simulink model "simulation"  (R2018b)
settings: Solver=ode4  StartTime=0.0  StopTime=200  FixedStep=0.001  RelTol=1e-3
model workspace: external: MAT-File Y:\Aerospace\AeroSpace 4\Term 2\AutoPilot (Dr. Osama Saaid)\Tasks\Task 7\code\Non-Linear Simulation\AC_data.mat (data not in the file)
values from neighbouring files (symbols this model uses):
  stability_matrix = [-0.0415 0 -0.162 0 -0.00076 0 0 -0.338 0 0 0 0 ... (72 elements, 6x12)]    [AC_data.mat]
undefined symbols (not defined in the file or in its folder): plane, rotationVectorToMatrix, servo
libraries: simulink_extras x12, cstblocks x3, shared6dof x1, dspsigops x1
settings Model: Creator=OWNER  LastModifiedBy=OWNER

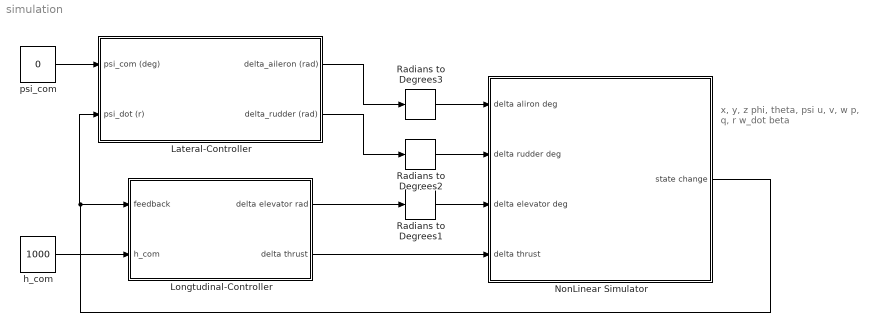
== system simulation ==
  note: x, y, z
      |
      | phi, theta, psi
      |
      | u, v, w
      |
      | p, q, r
      |
      | w_dot
      |
      | beta
  Lateral-Controller : Subsystem
  Longtudinal-Controller : Subsystem
  NonLinear Simulator : Subsystem
  Radians to Degrees1 : simulink_extras/Transformations/Radians to Degrees
  Radians to Degrees2 : simulink_extras/Transformations/Radians to Degrees
  Radians to Degrees3 : simulink_extras/Transformations/Radians to Degrees
  h_com : Constant  Value=1000
  psi_com : Constant  Value=0
  wires:
  Radians to Degrees3/1 -> NonLinear Simulator/1(delta aliron deg)
  Radians to Degrees2/1 -> NonLinear Simulator/2(delta rudder deg)
  Radians to Degrees1/1 -> NonLinear Simulator/3(delta elevator deg)
  h_com/1 -> Longtudinal-Controller/2(h_com)
  Longtudinal-Controller/1(delta elevator rad) -> Radians to Degrees1/1
  Longtudinal-Controller/2(delta thrust) -> NonLinear Simulator/4(delta thrust)
  psi_com/1 -> Lateral-Controller/1(psi_com (deg))
  Lateral-Controller/1(delta_aileron (rad)) -> Radians to Degrees3/1
  Lateral-Controller/2(delta_rudder (rad)) -> Radians to Degrees2/1
  NonLinear Simulator/1(state change) -> Lateral-Controller/2(psi_dot (r)), Longtudinal-Controller/1(feedback)

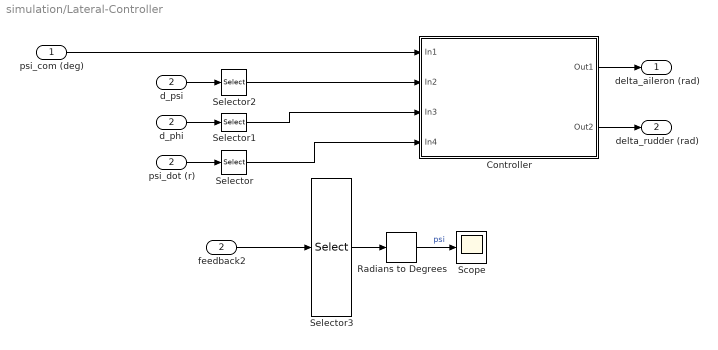
== system simulation/Lateral-Controller ==
  psi_com (deg) : Inport
  psi_dot (r) : Inport  Port=2
  Controller : Subsystem
  Radians to Degrees : simulink_extras/Transformations/Radians to Degrees
  Scope : Scope
  Selector : Selector  InputPortWidth=14  IndexOptions=Index vector (dialog)  Indices=[12]  OutputSizes=1
  Selector1 : Selector  InputPortWidth=14  IndexOptions=Index vector (dialog)  Indices=[4]  OutputSizes=1
  Selector2 : Selector  InputPortWidth=14  IndexOptions=Index vector (dialog)  Indices=[6]  OutputSizes=1
  Selector3 : Selector  InputPortWidth=14  IndexOptions=Index vector (dialog)  Indices=[6]  OutputSizes=1
  d_phi : InportShadow  Port=2
  d_psi : InportShadow  Port=2
  feedback2 : InportShadow  Port=2
  delta_aileron (rad) : Outport  VectorParamsAs1DForOutWhenUnconnected=on
  delta_rudder (rad) : Outport  Port=2  VectorParamsAs1DForOutWhenUnconnected=on
  wires:
  psi_com (deg)/1 -> Controller/1(In1)
  d_psi/1 -> Selector2/1
  d_phi/1 -> Selector1/1
  psi_dot (r)/1 -> Selector/1
  Controller/1(Out1) -> delta_aileron (rad)/1
  Controller/2(Out2) -> delta_rudder (rad)/1
  Selector3/1 -> Radians to Degrees/1
  feedback2/1 -> Selector3/1
  Radians to Degrees/1 -> Scope/1  "psi"
  Selector2/1 -> Controller/2(In2)
  Selector1/1 -> Controller/3(In3)
  Selector/1 -> Controller/4(In4)

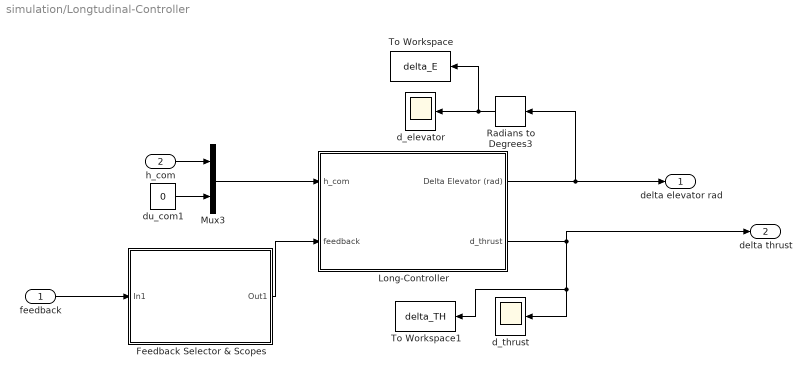
== system simulation/Longtudinal-Controller ==
  feedback : Inport
  h_com : Inport  Port=2
  Feedback Selector & Scopes : Subsystem
  "Long-Controller " : Subsystem
  Mux3 : Mux  Inputs=2
  Radians to Degrees3 : simulink_extras/Transformations/Radians to Degrees
  To Workspace : ToWorkspace  VariableName=delta_E  SaveFormat=Timeseries  SampleTime=-1
  To Workspace1 : ToWorkspace  VariableName=delta_TH  SaveFormat=Timeseries  SampleTime=-1
  d_elevator : Scope
  d_thrust : Scope
  du_com1 : Constant  Value=0
  delta elevator rad : Outport
  delta thrust : Outport  Port=2
  wires:
  Feedback Selector & Scopes/1(Out1) -> "Long-Controller "/2(feedback)
  Mux3/1 -> "Long-Controller "/1(h_com)
  h_com/1 -> Mux3/1
  du_com1/1 -> Mux3/2
  "Long-Controller "/1(Delta Elevator (rad)) -> delta elevator rad/1, Radians to Degrees3/1
  feedback/1 -> Feedback Selector & Scopes/1(In1)
  Radians to Degrees3/1 -> To Workspace/1, d_elevator/1
  "Long-Controller "/2(d_thrust) -> delta thrust/1, To Workspace1/1, d_thrust/1

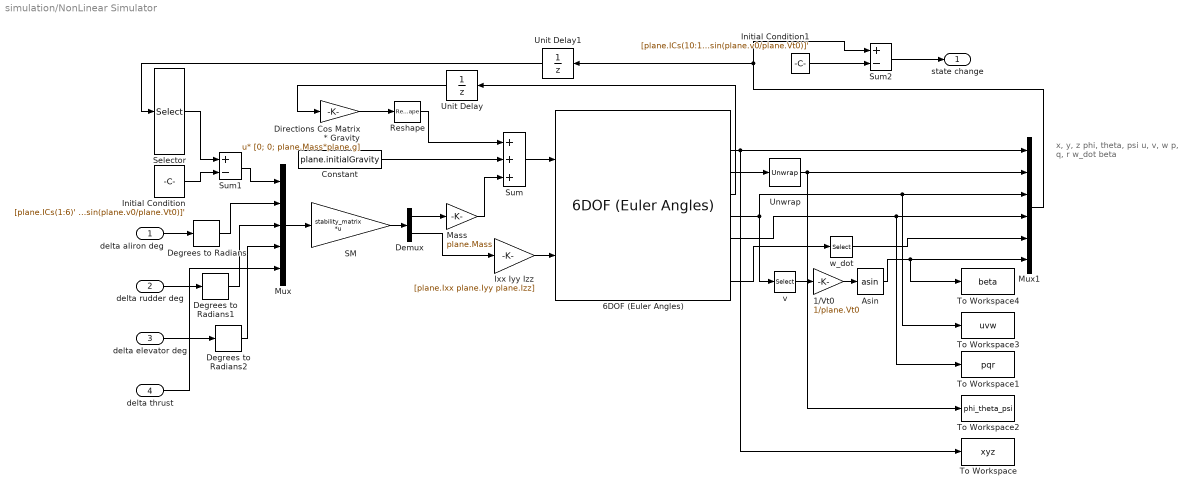
== system simulation/NonLinear Simulator ==
  note: x, y, z
      |
      | phi, theta, psi
      |
      | u, v, w
      |
      | p, q, r
      |
      | w_dot
      |
      | beta
  delta aliron deg : Inport
  delta rudder deg : Inport  Port=2
  delta elevator deg : Inport  Port=3
  delta thrust : Inport  Port=4
  1/Vt0 : Gain  Gain=1/plane.Vt0
  6DOF (Euler Angles) : shared6dof/6DOF (Euler Angles)  units=English (Velocity in ft/s)  mtype=Fixed  rep=Euler Angles  xme_0=[plane.ICs(10:12) ]'  Vm_0=[plane.ICs(1:3)]'  eul_0=[plane.ICs(7:9)]'  pm_0=[plane.ICs(4:6)]'  mass_0=plane.Mass  mass_e=0.5  mass_f=2.0  inertia=plane.I  inertia_e=eye(3)  inertia_f=2*eye(3)  k_quat=1.0  vre_flag=on  abi_flag=off  aMode=0  xme_statename=''  Vm_statename=''  eul_statename=''  quat_statename=''  pm_statename=''  mass_statename=''
      settings: SourceProductBaseCode=AE
  Asin : Trigonometry  Operator=asin
  Constant : Constant  Value=plane.initialGravity
  Degrees to Radians : simulink_extras/Transformations/Degrees to Radians
  Degrees to Radians1 : simulink_extras/Transformations/Degrees to Radians
  Degrees to Radians2 : simulink_extras/Transformations/Degrees to Radians
  Demux : Demux  Outputs=2
  Directions Cos Matrix * Gravity : Gain  Gain=[0; 0; plane.Mass*plane.g]  Multiplication=Matrix(u*K)
  Initial Condition : Constant  Value=[plane.ICs(1:6)' plane.ICs_dot0(3)' asin(plane.v0/plane.Vt0)]'
  Initial Condition1 : Constant  Value="[plane.ICs(10:12)' plane.ICs(7:9)' plane.ICs(1:6)'  plane.ICs_dot0(3)' asin(plane.v0/plane.Vt0)]'"
  Ixx Iyy Izz : Gain  Gain=[plane.Ixx plane.Iyy plane.Izz]
  "Mass " : Gain  Gain=plane.Mass
  Mux : Mux  Inputs=5
  Mux1 : Mux  Inputs=6
  Reshape : Reshape
  SM : Gain  Gain=stability_matrix  Multiplication=Matrix(K*u) (u vector)
  Selector : Selector  InputPortWidth=14  IndexOptions=Index vector (dialog)  Indices=[7:14]  OutputSizes=1
  Sum : Sum  Inputs=+++
  Sum1 : Sum  Inputs=+-
  Sum2 : Sum  Inputs=+-
  To Workspace : ToWorkspace  VariableName=xyz  SaveFormat=Timeseries  SampleTime=-1
  To Workspace1 : ToWorkspace  VariableName=pqr  SaveFormat=Timeseries  SampleTime=-1
  To Workspace2 : ToWorkspace  VariableName=phi_theta_psi  SaveFormat=Timeseries  SampleTime=-1
  To Workspace3 : ToWorkspace  VariableName=uvw  SaveFormat=Timeseries  SampleTime=-1
  To Workspace4 : ToWorkspace  VariableName=beta  SaveFormat=Timeseries  SampleTime=-1
  Unit Delay : UnitDelay  InitialCondition=rotationVectorToMatrix(plane.ICs(7:9))  SampleTime=-1
  Unit Delay1 : UnitDelay  InitialCondition=[plane.ICs(10:12)' plane.ICs(7:9)' plane.ICs(1:3)' plane.ICs(4:6)' plane.ICs_dot0(3) asin(plane.v0/plane.Vt0)]'  SampleTime=-1
  Unwrap : dspsigops/Unwrap  tol=pi  running=off
  v : Selector  InputPortWidth=3  IndexOptions=Index vector (dialog)  Indices=[2]  OutputSizes=1
  w_dot : Selector  InputPortWidth=3  IndexOptions=Index vector (dialog)  Indices=[3]  OutputSizes=1
  state change : Outport
  wires:
  Mux1/1 -> Sum2/1, Unit Delay1/1
  6DOF (Euler Angles)/2 -> Mux1/1, To Workspace/1
  "Mass "/1 -> Sum/3
  Constant/1 -> Sum/2
  1/Vt0/1 -> Asin/1
  Demux/1 -> "Mass "/1
  Sum/1 -> 6DOF (Euler Angles)/1
  6DOF (Euler Angles)/5 -> v/1, To Workspace3/1, Mux1/3
  6DOF (Euler Angles)/6 -> To Workspace1/1, Mux1/4
  Unit Delay/1 -> Directions Cos Matrix * Gravity/1
  Degrees to Radians1/1 -> Mux/3
  delta elevator deg/1 -> Degrees to Radians2/1
  6DOF (Euler Angles)/4 -> Unit Delay/1
  Directions Cos Matrix * Gravity/1 -> Reshape/1
  Reshape/1 -> Sum/1
  6DOF (Euler Angles)/8 -> w_dot/1
  6DOF (Euler Angles)/3 -> Unwrap/1
  Selector/1 -> Sum1/1
  Degrees to Radians/1 -> Mux/2
  Asin/1 -> Mux1/6, To Workspace4/1
  Degrees to Radians2/1 -> Mux/4
  Mux/1 -> SM/1
  Ixx Iyy Izz/1 -> 6DOF (Euler Angles)/2
  delta aliron deg/1 -> Degrees to Radians/1
  delta thrust/1 -> Mux/5
  v/1 -> 1/Vt0/1
  Initial Condition/1 -> Sum1/2
  Unit Delay1/1 -> Selector/1
  Sum1/1 -> Mux/1
  w_dot/1 -> Mux1/5
  SM/1 -> Demux/1
  Demux/2 -> Ixx Iyy Izz/1
  delta rudder deg/1 -> Degrees to Radians1/1
  Unwrap/1 -> Mux1/2, To Workspace2/1
  Initial Condition1/1 -> Sum2/2
  Sum2/1 -> state change/1

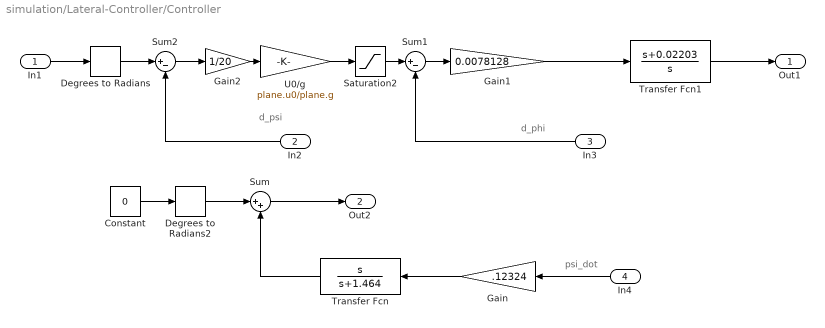
== system simulation/Lateral-Controller/Controller ==
  note: psi_dot
  note: d_psi
  note: d_phi
  In1 : Inport
  In2 : Inport  Port=2
  In3 : Inport  Port=3
  In4 : Inport  Port=4
  Constant : Constant  Value=0
  Degrees to Radians : simulink_extras/Transformations/Degrees to Radians
  Degrees to Radians2 : simulink_extras/Transformations/Degrees to Radians
  Gain : Gain  Gain=.12324
  Gain1 : Gain  Gain=0.0078128
  Gain2 : Gain  Gain=1/20
  Saturation2 : Saturate  UpperLimit=30*pi/180  LowerLimit=-30*pi/180
  Sum : Sum  Inputs=|++
  Sum1 : Sum  Inputs=|+-
  Sum2 : Sum  Inputs=|+-
  Transfer Fcn : TransferFcn  Numerator=[1 0]  Denominator=[1 1.464]
  Transfer Fcn1 : TransferFcn  Numerator=[1 0.02203]  Denominator=[1 0]
  U0/g : Gain  Gain=plane.u0/plane.g
  Out1 : Outport
  Out2 : Outport  Port=2
  wires:
  Degrees to Radians/1 -> Sum2/1
  Gain/1 -> Transfer Fcn/1
  In2/1 -> Sum2/2
  Transfer Fcn/1 -> Sum/2
  Degrees to Radians2/1 -> Sum/1
  Sum2/1 -> Gain2/1
  In4/1 -> Gain/1
  In3/1 -> Sum1/2
  In1/1 -> Degrees to Radians/1
  Saturation2/1 -> Sum1/1
  Sum1/1 -> Gain1/1
  U0/g/1 -> Saturation2/1
  Gain2/1 -> U0/g/1
  Constant/1 -> Degrees to Radians2/1
  Gain1/1 -> Transfer Fcn1/1
  Sum/1 -> Out2/1
  Transfer Fcn1/1 -> Out1/1

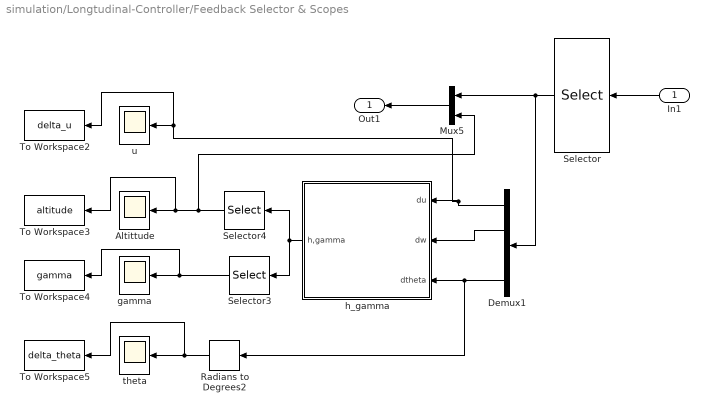
== system simulation/Longtudinal-Controller/Feedback Selector & Scopes ==
  In1 : Inport
  Altittude : Scope
  Demux1 : Demux
  Mux5 : Mux  Inputs=2
  Radians to Degrees2 : simulink_extras/Transformations/Radians to Degrees
  Selector : Selector  InputPortWidth=14  IndexOptions=Index vector (dialog)  Indices=[7 9 11 5]  OutputSizes=1
  Selector3 : Selector  InputPortWidth=2  IndexOptions=Index vector (dialog)  Indices=[2]  OutputSizes=1
  Selector4 : Selector  InputPortWidth=2  IndexOptions=Index vector (dialog)  Indices=[1]  OutputSizes=1
  To Workspace2 : ToWorkspace  VariableName=delta_u  SaveFormat=Timeseries  SampleTime=-1
  To Workspace3 : ToWorkspace  VariableName=altitude  SaveFormat=Timeseries  SampleTime=-1
  To Workspace4 : ToWorkspace  VariableName=gamma  SaveFormat=Timeseries  SampleTime=-1
  To Workspace5 : ToWorkspace  VariableName=delta_theta  SaveFormat=Timeseries  SampleTime=-1
  gamma : Scope
  h_gamma : Subsystem
  theta : Scope
  u : Scope
  Out1 : Outport
  wires:
  Selector/1 -> Demux1/1, Mux5/1
  Demux1/2 -> h_gamma/2(dw)
  Demux1/1 -> To Workspace2/1, u/1, h_gamma/1(du)
  Selector4/1 -> Mux5/2, To Workspace3/1, Altittude/1
  h_gamma/1(h,gamma) -> Selector3/1, Selector4/1
  Selector3/1 -> To Workspace4/1, gamma/1
  Demux1/4 -> Radians to Degrees2/1, h_gamma/3(dtheta)
  Radians to Degrees2/1 -> To Workspace5/1, theta/1
  In1/1 -> Selector/1
  Mux5/1 -> Out1/1

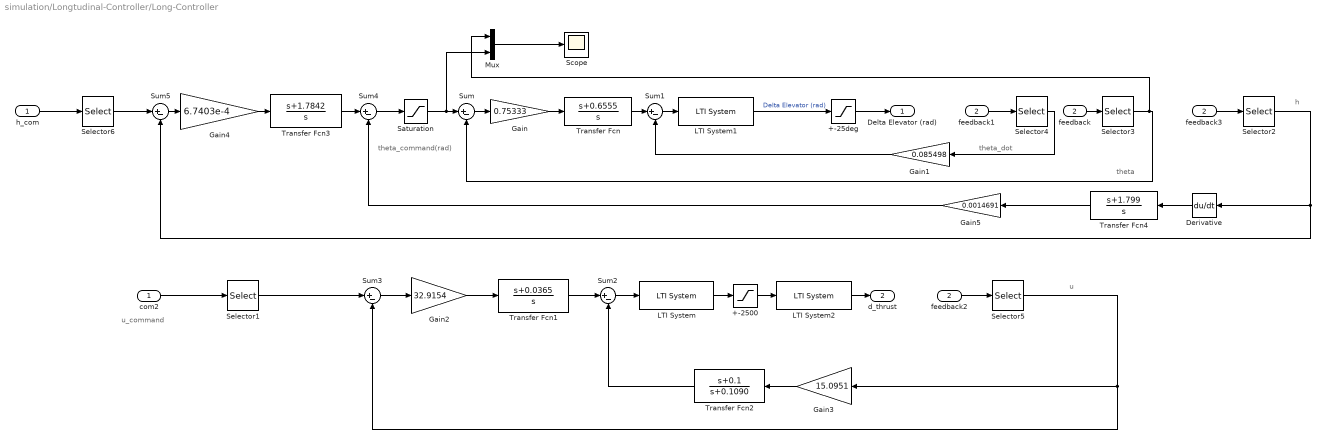
== system simulation/Longtudinal-Controller/Long-Controller  ==
  note: u_command
  note: u
  note: theta
  note: theta_command(rad)
  note: theta_dot
  note: h
  h_com : Inport
  feedback : Inport  Port=2
  +-2500 : Saturate  UpperLimit=2500  LowerLimit=-2500
  +-25deg : Saturate  UpperLimit=25*pi/180  LowerLimit=-25*pi/180
  Derivative : Derivative
  Gain : Gain  Gain=0.75333
  Gain1 : Gain  Gain=0.085498
  Gain2 : Gain  Gain=32.9154
  Gain3 : Gain  Gain=15.0951
  Gain4 : Gain  Gain=6.7403e-4
  Gain5 : Gain  Gain=0.0014691
  LTI System : cstblocks/LTI System  sys=servo  IC=[]
  LTI System1 : cstblocks/LTI System  sys=-servo  IC=[]
  LTI System2 : cstblocks/LTI System  sys=engine_timelag  IC=[]
  Mux : Mux  Inputs=2
  Saturation : Saturate  LowerLimit=-.5
  Scope : Scope
  Selector1 : Selector  InputPortWidth=2  IndexOptions=Index vector (dialog)  Indices=[2]  OutputSizes=1
  Selector2 : Selector  InputPortWidth=5  IndexOptions=Index vector (dialog)  Indices=[5]  OutputSizes=1
  Selector3 : Selector  InputPortWidth=5  IndexOptions=Index vector (dialog)  Indices=[4]  OutputSizes=1
  Selector4 : Selector  InputPortWidth=5  IndexOptions=Index vector (dialog)  Indices=[3]  OutputSizes=1
  Selector5 : Selector  InputPortWidth=5  IndexOptions=Index vector (dialog)  Indices=[1]  OutputSizes=1
  Selector6 : Selector  InputPortWidth=2  IndexOptions=Index vector (dialog)  Indices=[1]  OutputSizes=1
  Sum{,1..5} (6 alike) : Sum  Inputs=|+-
  Transfer Fcn : TransferFcn  Numerator=[1 +0.6555]  Denominator=[1 0]
  Transfer Fcn1 : TransferFcn  Numerator=[1 0.0365]  Denominator=[1 0]
  Transfer Fcn2 : TransferFcn  Numerator=[1 0.1]  Denominator=[1 0.1090]
  Transfer Fcn3 : TransferFcn  Numerator=[1 1.7842]  Denominator=[1 0]
  Transfer Fcn4 : TransferFcn  Numerator=[1 +1.799]  Denominator=[1 0]
  com2 : InportShadow
  feedback1 : InportShadow  Port=2
  feedback2 : InportShadow  Port=2
  feedback3 : InportShadow  Port=2
  Delta Elevator (rad) : Outport  VectorParamsAs1DForOutWhenUnconnected=on
  d_thrust : Outport  Port=2  VectorParamsAs1DForOutWhenUnconnected=on
  wires:
  Transfer Fcn/1 -> Sum1/1
  Gain/1 -> Transfer Fcn/1
  Gain1/1 -> Sum1/2
  Sum1/1 -> LTI System1/1
  Sum/1 -> Gain/1
  LTI System1/1 -> +-25deg/1  "Delta Elevator (rad)"
  Selector3/1 -> Mux/1, Sum/2
  LTI System/1 -> +-2500/1
  Sum2/1 -> LTI System/1
  Selector5/1 -> Gain3/1, Sum3/2
  Transfer Fcn1/1 -> Sum2/1
  Gain3/1 -> Transfer Fcn2/1
  Gain2/1 -> Transfer Fcn1/1
  Transfer Fcn2/1 -> Sum2/2
  Sum3/1 -> Gain2/1
  com2/1 -> Selector1/1
  Selector1/1 -> Sum3/1
  feedback1/1 -> Selector4/1
  feedback/1 -> Selector3/1
  Selector4/1 -> Gain1/1
  LTI System2/1 -> d_thrust/1
  feedback2/1 -> Selector5/1
  Sum5/1 -> Gain4/1
  Sum4/1 -> Saturation/1
  feedback3/1 -> Selector2/1
  Selector2/1 -> Derivative/1, Sum5/2
  h_com/1 -> Selector6/1
  Selector6/1 -> Sum5/1
  Gain4/1 -> Transfer Fcn3/1
  Transfer Fcn3/1 -> Sum4/1
  Gain5/1 -> Sum4/2
  Transfer Fcn4/1 -> Gain5/1
  Derivative/1 -> Transfer Fcn4/1
  Mux/1 -> Scope/1
  Saturation/1 -> Mux/2, Sum/1
  +-2500/1 -> LTI System2/1
  +-25deg/1 -> Delta Elevator (rad)/1

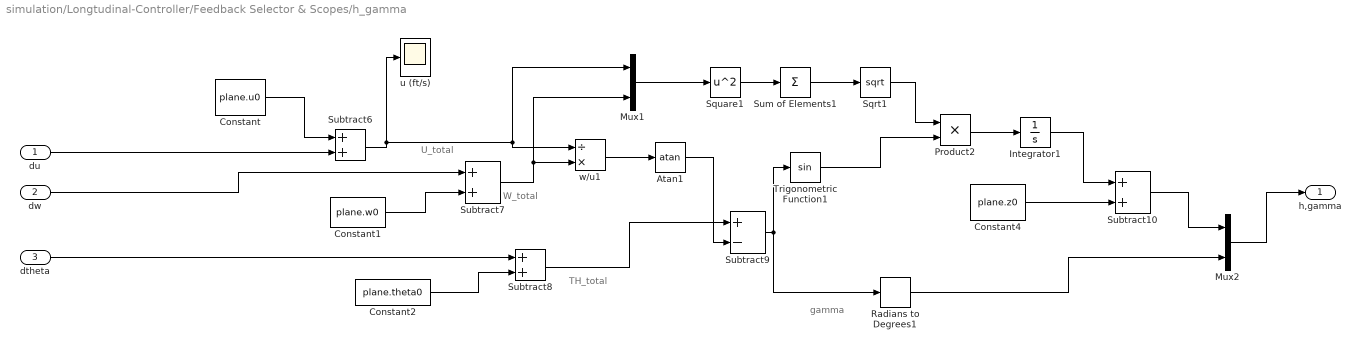
== system simulation/Longtudinal-Controller/Feedback Selector & Scopes/h_gamma ==
  note: U_total
  note: W_total
  note: TH_total
  note: gamma
  du : Inport
  dw : Inport  Port=2
  dtheta : Inport  Port=3
  Atan1 : Trigonometry  Operator=atan
  Constant : Constant  Value=plane.u0
  Constant1 : Constant  Value=plane.w0
  Constant2 : Constant  Value=plane.theta0  VectorParams1D=off
  Constant4 : Constant  Value=plane.z0
  Integrator1 : Integrator
  Mux1 : Mux  Inputs=2
  Mux2 : Mux  Inputs=2
  Product2 : Product
  Radians to Degrees1 : simulink_extras/Transformations/Radians to Degrees
  Sqrt1 : Sqrt  SaturateOnIntegerOverflow=on
  Square1 : Math  Operator=square  SaturateOnIntegerOverflow=on
  Subtract{6..8,10} (4 alike) : Sum
  Subtract9 : Sum  Inputs=+-
  Sum of Elements1 : Sum  Inputs=+
  Trigonometric Function1 : Trigonometry
  u (ft/s) : Scope
  w/u1 : Product  Inputs=/*
  h,gamma : Outport
  wires:
  Constant4/1 -> Subtract10/2
  w/u1/1 -> Atan1/1
  Subtract7/1 -> w/u1/2, Mux1/2
  Constant1/1 -> Subtract7/2
  Square1/1 -> Sum of Elements1/1
  Radians to Degrees1/1 -> Mux2/2
  Subtract8/1 -> Subtract9/1
  Constant/1 -> Subtract6/1
  Subtract9/1 -> Trigonometric Function1/1, Radians to Degrees1/1
  Sum of Elements1/1 -> Sqrt1/1
  Trigonometric Function1/1 -> Product2/2
  Constant2/1 -> Subtract8/2
  du/1 -> Subtract6/2
  dtheta/1 -> Subtract8/1
  Sqrt1/1 -> Product2/1
  dw/1 -> Subtract7/1
  Subtract6/1 -> u (ft/s)/1, w/u1/1, Mux1/1
  Integrator1/1 -> Subtract10/1
  Mux1/1 -> Square1/1
  Product2/1 -> Integrator1/1
  Atan1/1 -> Subtract9/2
  Subtract10/1 -> Mux2/1
  Mux2/1 -> h,gamma/1
